simulink model "FSK_modelo"  (R2020b)
settings: Solver=VariableStepAuto  StartTime=0.0  StopTime=205*6  RelTol=1e-3
values from neighbouring files (symbols this model uses):
  Pd = 40    [simulacion_qam.m]    (also in simulacioon.m)
libraries: commsynccomp2 x1
settings Model: Creator=Mateo  LastModifiedBy=Mateo
settings DataIOCC: ReturnWorkspaceOutputs=off

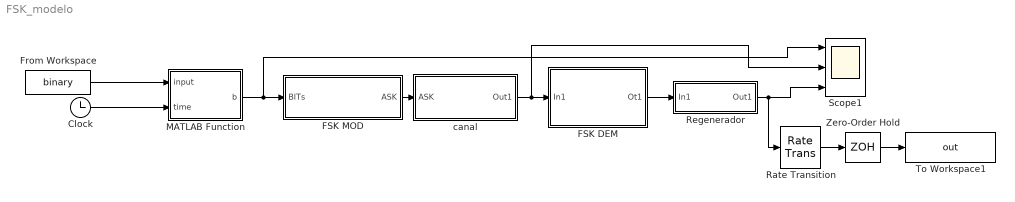
== system FSK_modelo ==
  Clock : Clock
  FSK DEM : Subsystem
  FSK MOD : Subsystem
  From Workspace : FromWorkspace  VariableName=binary
  MATLAB Function : MATLAB Function  TreatAsAtomicUnit=on
  Rate Transition : RateTransition
  Regenerador : Subsystem
  Scope1 : Scope  NumInputPorts=3
  To Workspace1 : ToWorkspace  VariableName=out  SaveFormat=Timeseries  SampleTime=-1
  Zero-Order Hold : ZeroOrderHold  SampleTime=6
  canal : Subsystem
  wires:
  FSK DEM/1(Ot1) -> Regenerador/1(In1)
  FSK MOD/1(ASK) -> canal/1(ASK)
  Regenerador/1(Out1) -> Rate Transition/1, Scope1/3
  canal/1(Out1) -> Scope1/2, FSK DEM/1(In1)
  Clock/1 -> MATLAB Function/2(time)
  From Workspace/1 -> MATLAB Function/1(input)
  MATLAB Function/1(b) -> FSK MOD/1(BITs), Scope1/1
  Rate Transition/1 -> Zero-Order Hold/1
  Zero-Order Hold/1 -> To Workspace1/1

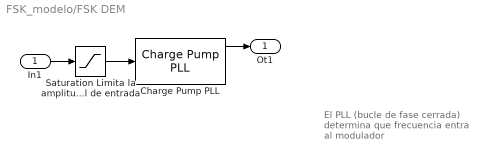
== system FSK_modelo/FSK DEM ==
  note: El PLL (bucle de fase cerrada)
      | determina que frecuencia
      | entra al modulador
  In1 : Inport
  Charge Pump PLL : commsynccomp2/Charge Pump PLL  Fn=[2*pi*1]  Fd="[1   2*pi*1]"  Kvco=4  Fc=10  Ph=0  Ac=1
      settings: SourceProductBaseCode=CM
  Saturation Limita la amplitud de la señal de entrada : Saturate
  Ot1 : Outport
  wires:
  In1/1 -> Saturation Limita la amplitud de la señal de entrada/1
  Charge Pump PLL/1 -> Ot1/1
  Saturation Limita la amplitud de la señal de entrada/1 -> Charge Pump PLL/1

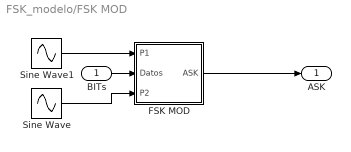
== system FSK_modelo/FSK MOD ==
  BITs : Inport
  FSK MOD : Subsystem
  Sine Wave : Sin  Frequency=2*pi*12  Samples=25  SampleTime=0.01
  Sine Wave1 : Sin  Frequency=2*pi*8  Samples=50  SampleTime=0.01
  ASK : Outport
  wires:
  BITs/1 -> FSK MOD/2(Datos)
  FSK MOD/1(ASK) -> ASK/1
  Sine Wave1/1 -> FSK MOD/1(P1)
  Sine Wave/1 -> FSK MOD/3(P2)

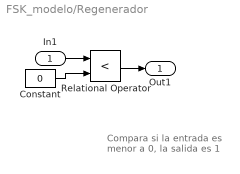
== system FSK_modelo/Regenerador ==
  note: Compara si la entrada
      | es menor a 0, la salida es 1
  In1 : Inport
  Constant : Constant  Value=0
  Relational Operator : RelationalOperator  Operator=<  OutDataTypeStr=boolean  RndMeth=Nearest
  Out1 : Outport
  wires:
  Relational Operator/1 -> Out1/1
  In1/1 -> Relational Operator/1
  Constant/1 -> Relational Operator/2

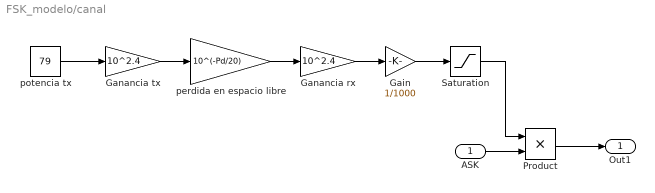
== system FSK_modelo/canal ==
  ASK : Inport
  Gain : Gain  Gain=1/1000
  Ganancia rx : Gain  Gain=10^2.4
  Ganancia tx : Gain  Gain=10^2.4
  Product : Product
  Saturation : Saturate  UpperLimit=1  LowerLimit=0
  perdida en espacio libre : Gain  Gain=10^(-Pd/20)
  potencia tx : Constant  Value=79
  Out1 : Outport
  wires:
  potencia tx/1 -> Ganancia tx/1
  Ganancia tx/1 -> perdida en espacio libre/1
  perdida en espacio libre/1 -> Ganancia rx/1
  Product/1 -> Out1/1
  Saturation/1 -> Product/1
  ASK/1 -> Product/2
  Ganancia rx/1 -> Gain/1
  Gain/1 -> Saturation/1

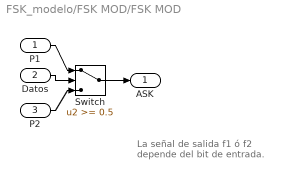
== system FSK_modelo/FSK MOD/FSK MOD ==
  note: La señal de salida f1 ó f2
      | depende del bit de entrada.
  P1 : Inport
  Datos : Inport  Port=2
  P2 : Inport  Port=3
  Switch : Switch  Threshold=0.5
  ASK : Outport
  wires:
  P1/1 -> Switch/1
  Datos/1 -> Switch/2
  Switch/1 -> ASK/1
  P2/1 -> Switch/3

== matlab function FSK_modelo/MATLAB Function ==
  data: input input; b output; time input
function b = fcn(input,time)
    b=input(floor(time/6)+1);
end
